simulink model "CM13_2024a_MachE_for_UA_HIL"  (R2024a)
settings: Solver=ode1  StartTime=0.0  StopTime=Inf  FixedStep=0.001  RelTol=1e-3  EnableMultiTasking=on
PreLoadFcn:
  | % if ~length(which('cmcmd')), cmenv; end
PostLoadFcn:
  | if any(exist('dsrtsu_mdlpostloadfcn', 'file') ~= 0), dsrtsu_mdlpostloadfcn('Execute', bdroot); end
InitFcn:
  | , if any(exist('rtifpga_mdlclblib', 'file') ~= 0), rtifpga_mdlclblib('Init', bdroot); end,
  | , if any(exist('dsmpb_private', 'file') ~= 0), dsmpb_private('dsmpb_mdlclblib', 'Init', bdroot); end,
values from neighbouring files (symbols this model uses):
  CoastDown =     [Run_Simulink.mat]
  limitedMCT =     [Run_Simulink.mat]
  MCT =     [Run_Simulink.mat]
  pMCT =     [Run_Simulink.mat]
  RealSimPara =     [Run_Simulink.mat]
  Ref_speed = [13 13.007895099 13.015778396 13.023649891 13.031509584 13.039357475 13.047193564 13.055017851 13.062830336 13.070631019 13.0784199 13.086196979 ... (2669 elements, 2669x1)]    [Ref_speed_and_time.mat]
  Ref_time = [0 0.01 0.02 0.03 0.04 0.05 0.06 0.07 0.08 0.09 0.1 0.11 ... (2669 elements, 2669x1)]    [Ref_speed_and_time.mat]
  US06 =     [Run_Simulink.mat]
undefined symbols (not defined in the file or in its folder): AccelCmd, ActTqLF_Nm_, ActTqLR_Nm_, ActTqRF_Nm_, ActTqRR_Nm_, BattChargeLimitMaxPwr, BattChargeLimitSocBpts, BattChargeLimitTbl, BattChrgCapcty, BattDischargeLimitSocBpts, BattDischargeLimitTbl, BattDischargeMaxPwr, BattNumCellsParallel, BattNumCellsSeries, BattOpenVoltCapBpts, BattOpenVoltTbl, BattResistSocBpts, BattResistTbl, BattResistTempBpts, BrakeMaxPrs, BrakeMaxTrq, ChassisDistCg2FrontAxle, ChassisDistCg2RearAxle, ChassisVehMass, CltchCmd, DecelCmd, DiffRatio, DiscIntNeverNeededParam, EnvGravCnst, EnvPrs, EnvTemp, FuelSpecificGrav, GearCmd, h, InitStates, lgSw, MtrEffSpdBpts, MtrEffTbl, MtrEffTrqBpts, MtrPwrMax, MtrTrqMax, planned_speed, planned_time, ref_speed, ref_time, rticanmm_blockfcn, rticanmm_initfcn, SteeringCmd, SupvsryCtrlRegenBrkCutOffTbl, SupvsryCtrlRegenSpdBpts, TestScnrioCycleNum, VEH
libraries: simulink x264, VSIGenLib x262, etargetslib x201, dsmpblib x161, CarMaker4SL x142, rtimmsu_dsrtlib x32, vehdynlibtire x24, autolibshared x19, vehdynlibsuspension x14, vehdynlibtirecommon x14, autolibutils x10, VsrLibWheel x8
(part 16 of 48)

== system CM13_2024a_MachE_for_UA_HIL/CarMaker_new/IPG Vehicle/Driver and Drive Cycle/Get Cycle Clock Time ==
  Cycle Trigger : Inport
  Add1 : Sum  Inputs=+-
  Clock1 : Clock
  Clock2 : Clock
  Data Type Conversion : DataTypeConversion  OutDataTypeStr=double  SaturateOnIntegerOverflow=off  RndMeth=Floor
  Memory4 : Memory
  Switch : Switch  Criteria=u2 > Threshold  SaturateOnIntegerOverflow=off  InputSameDT=off
  tCycle : Outport
  wires:
  Switch/1 -> Add1/2, Memory4/1
  Clock1/1 -> Add1/1
  Clock2/1 -> Switch/3
  Add1/1 -> tCycle/1  "tCycle"
  Memory4/1 -> Switch/1
  Cycle Trigger/1 -> Data Type Conversion/1
  Data Type Conversion/1 -> Switch/2

== system CM13_2024a_MachE_for_UA_HIL/CarMaker_new/IPG Vehicle/Driver and Drive Cycle/IDM ==
  note: In IPG, when the ego vehicle slipped side to side, it will ignore the front vehicle as in the path. The <RadarL> "detects nearest point in the path" , thus ego vehilce will no longer consider the front vehilce as "in path" and ACC/IDM will have incorrect output.
      |
      | Second object sensor <Backup> is added, it dectects nearest point, ensuring ego vehicle stopped at close range.
  CM_Time : Inport
  Add1 : Sum
  Add2 : Sum
  Add3 : Sum  Commented=on
  Bus Selector : BusSelector  OutputSignals=NearPnt ds x,NearPnt ds y,NearPnt dv x
  Bus Selector1 : BusSelector  OutputSignals=dtct
  Bus Selector2 : BusSelector  OutputSignals=dtct
  Bus Selector3 : BusSelector  OutputSignals=NearPnt ds x,NearPnt ds y
  Bus Selector4 : BusSelector  Commented=on  OutputSignals=NearPnt ds x,NearPnt ds y,NearPnt dv x
  Bus Selector5 : BusSelector  Commented=on  OutputSignals=dtct
  Bus Selector6 : BusSelector  OutputSignals=Dist,Vrel
  Compare To Constant : simulink/Logic and Bit Operations/Compare To Constant  relop=>=  const=30  OutDataTypeStr=boolean
  Constant : Constant  Value=0
  Constant1 : Constant  Value=99999
  Constant2 : Constant  Value=99999
  Dis2lead_Raw : Scope
  Math Function{,1..3} (4 alike) : Math  Operator=square
  Math Function4 : Math  Commented=on  Operator=square
  Math Function5 : Math  Commented=on  Operator=square
  ObjIndex : Scope
  Object Sensor 1 : CarMaker4SL/Sensors/Object Sensor  xname=RadarS  xstime=Continuous
      settings: SourceProductName=CarMaker4SL
  Object Sensor 2 : CarMaker4SL/Sensors/Object Sensor  xname=RadarL  xstime=Continuous
      settings: SourceProductName=CarMaker4SL
  Object Sensor Object : CarMaker4SL/Sensors/Object Sensor Object  Commented=on  xname=RadarL  ximode=Observed Objects  xstime=Continuous
      settings: SourceProductName=CarMaker4SL
  Object Sensor Object 1 : CarMaker4SL/Sensors/Object Sensor Object  xname=INPORT  ximode=Observed Objects  xstime=Continuous
      settings: SourceProductName=CarMaker4SL
  Object Sensor Object 2 : CarMaker4SL/Sensors/Object Sensor Object  xname=INPORT  ximode=Observed Objects  xstime=Continuous
      settings: SourceProductName=CarMaker4SL
  Radar Sensor : CarMaker4SL/Sensors/Radar Sensor  xname=RadarReal  xstime=Continuous
      settings: SourceProductName=CarMaker4SL
  Radar Sensor Object : CarMaker4SL/Sensors/Radar Sensor Object  xname=INPORT  ximode=Observed Objects  xstime=Continuous
      settings: SourceProductName=CarMaker4SL
  Read CM Dict1 : CarMaker4SL/Read CM Dict  xname=Car.v  xsync=off  xstime=Continuous
  Scope1 : Scope  Commented=on
  Scope2 : Scope  Commented=on
  Scope3 : Scope
  Scope4 : Scope
  Square Root : Sqrt
  Square Root1 : Sqrt
  Square Root2 : Sqrt  Commented=on
  Subsystem : Subsystem
  Switch1 : Switch  Criteria=u2 > Threshold  SaturateOnIntegerOverflow=off  InputSameDT=off
  ego_ref_spd_m/s : Outport
  wires:
  Add1/1 -> Square Root/1
  Bus Selector1/1 -> Subsystem/1(is_detected)  "<dtct>"
  Bus Selector/3 -> Subsystem/4(rel_front_spd_m/s)  "<NearPnt dv x>"
  Object Sensor Object 2/3 -> Bus Selector1/1
  Read CM Dict1/1 -> Subsystem/2(ego_spd_m/s)  "VehSpd"
  Math Function/1 -> Add1/1
  Object Sensor Object 2/5 -> Bus Selector/1
  Math Function1/1 -> Add1/2
  Object Sensor 2/1 -> Object Sensor Object 2/1
  Constant2/1 -> Object Sensor Object 2/2
  Bus Selector/1 -> Math Function/1  "<NearPnt ds x>"
  Bus Selector/2 -> Math Function1/1  "<NearPnt ds y>"
  Subsystem/1(ego_ref_spd_m/s) -> Switch1/1
  Object Sensor 1/1 -> Object Sensor Object 1/1
  Constant1/1 -> Object Sensor Object 1/2
  Object Sensor Object 1/3 -> Bus Selector2/1
  Bus Selector2/1 -> Subsystem/5(backup_detected)  "<dtct>"
  CM_Time/1 -> [CM_Time]
  Compare To Constant/1 -> Switch1/2
  Constant/1 -> Switch1/3
  Switch1/1 -> ego_ref_spd_m/s/1
  [CM_Time] -> Compare To Constant/1
  Object Sensor Object 1/5 -> Bus Selector3/1
  Math Function3/1 -> Add2/2
  Math Function2/1 -> Add2/1
  Add2/1 -> Square Root1/1
  Bus Selector3/1 -> Math Function2/1  "<NearPnt ds x>"
  Bus Selector3/2 -> Math Function3/1  "<NearPnt ds y>"
  Bus Selector4/2 -> Math Function5/1  "<NearPnt ds y>"
  Bus Selector4/1 -> Math Function4/1  "<NearPnt ds x>"
  Object Sensor Object/3 -> Bus Selector5/1
  Object Sensor Object/5 -> Bus Selector4/1
  Square Root2/1 -> Scope1/1
  Bus Selector4/3 -> Scope2/1  "<NearPnt dv x>"
  Add3/1 -> Square Root2/1
  Math Function4/1 -> Add3/1
  Math Function5/1 -> Add3/2
  Square Root1/1 -> Subsystem/6(front_obj_dist_m)
  Square Root/1 -> Subsystem/3(int_veh_dist_m), Dis2lead_Raw/1
  Radar Sensor/1 -> Radar Sensor Object/1
  Radar Sensor Object/2 -> Bus Selector6/1
  Bus Selector6/1 -> Scope3/1  "<Dist>"
  Bus Selector6/2 -> Scope4/1  "<Vrel>"
  Object Sensor Object 2/1 -> ObjIndex/1

== system CM13_2024a_MachE_for_UA_HIL/CarMaker_new/IPG Vehicle/Mach-E CAN BM/Subsystem ==
  note: softRCM ECU
  Bus Creator : BusCreator  Inputs=5
  Logic : Subsystem
  Noise Generators : Subsystem  Commented=on
  Read CM Dict : CarMaker4SL/Read CM Dict  xname=Car.RollVel  xsync=off  xstime=Continuous
  Read CM Dict1 : CarMaker4SL/Read CM Dict  xname=Car.YawRate  xsync=off  xstime=Continuous
  Read CM Dict2 : CarMaker4SL/Read CM Dict  xname=Car.ax  xsync=off  xstime=Continuous
  Read CM Dict3 : CarMaker4SL/Read CM Dict  xname=Car.ay  xsync=off  xstime=Continuous
  Read CM Dict4 : CarMaker4SL/Read CM Dict  xname=Car.az  xsync=off  xstime=Continuous
  AccelYaw_out : Outport
  wires:
  Logic/1(Out1) -> AccelYaw_out/1
  Bus Creator/1 -> Logic/1(In1)
  Read CM Dict4/1 -> Bus Creator/5  "a_z_Vehicle_CoG_withG[m|s2]"
  Read CM Dict3/1 -> Bus Creator/4  "a_y_Vehicle_CoG_withG[m|s2]"
  Read CM Dict2/1 -> Bus Creator/3  "a_x_Vehicle_CoG_withG[m|s2]"
  Read CM Dict/1 -> Bus Creator/1  "RollRate_Vehicle_CoG[rad|s]"
  Read CM Dict1/1 -> Bus Creator/2  "YawRate_Vehicle_CoG[rad|s]"

== system CM13_2024a_MachE_for_UA_HIL/CarMaker_new/IPG Vehicle/Mach-E CAN BM/Subsystem1 ==
  note: softRCM ECU
  Roll : Inport
  Yaw : Inport  Port=2
  A_x : Inport  Port=3
  A_y : Inport  Port=4
  A_z : Inport  Port=5
  Add{,1..4} (5 alike) : Sum
  Bus Creator : BusCreator  Inputs=5
  Logic : Subsystem
  Noise Generators : Subsystem  Commented=on
  Read CM Dict : CarMaker4SL/Read CM Dict  xname=Car.RollVel  xsync=off  xstime=Continuous
  Read CM Dict1 : CarMaker4SL/Read CM Dict  xname=Car.YawRate  xsync=off  xstime=Continuous
  Read CM Dict2 : CarMaker4SL/Read CM Dict  xname=Car.ax  xsync=off  xstime=Continuous
  Read CM Dict3 : CarMaker4SL/Read CM Dict  xname=Car.ay  xsync=off  xstime=Continuous
  Read CM Dict4 : CarMaker4SL/Read CM Dict  xname=Car.az  xsync=off  xstime=Continuous
  AccelYaw_out : Outport
  wires:
  Add/1 -> Bus Creator/5  "a_z_Vehicle_CoG_withG[m|s2]"
  Add2/1 -> Bus Creator/3  "a_x_Vehicle_CoG_withG[m|s2]"
  Add4/1 -> Bus Creator/2  "YawRate_Vehicle_CoG[rad|s]"
  Add1/1 -> Bus Creator/4  "a_y_Vehicle_CoG_withG[m|s2]"
  Add3/1 -> Bus Creator/1  "RollRate_Vehicle_CoG[rad|s]"
  Logic/1(Out1) -> AccelYaw_out/1
  Bus Creator/1 -> Logic/1(In1)
  Read CM Dict4/1 -> Add/1  "a_z_Vehicle_CoG_withG[m|s2]"
  Read CM Dict3/1 -> Add1/1  "a_y_Vehicle_CoG_withG[m|s2]"
  Read CM Dict2/1 -> Add2/1  "a_x_Vehicle_CoG_withG[m|s2]"
  Read CM Dict/1 -> Add3/1  "RollRate_Vehicle_CoG[rad|s]"
  Read CM Dict1/1 -> Add4/1  "YawRate_Vehicle_CoG[rad|s]"
  Yaw/1 -> Add4/2
  A_x/1 -> Add2/2
  A_y/1 -> Add1/2
  Roll/1 -> Add3/2
  A_z/1 -> Add/2

== system CM13_2024a_MachE_for_UA_HIL/CarMaker_new/IPG Vehicle/MachE CAN/RTICANMM Gateway ==
  Enable : Inport
  DSRT Data Hook1 : rtimmsu_dsrtlib/Data Hook  ControllerName=RCM_ECU  PortID=RTICANMMRCM_ECU  BlockSet=can  blockdata=struct('version','1.0')
  DSRT Data Hook2 : rtimmsu_dsrtlib/Data Hook  ControllerName=RCM_Harness  PortID=RTICANMMRCM_Harness  BlockSet=can  blockdata=struct('version','1.0')
  ModelClose : Subsystem  mask(RTICANMMModelClose){}
  TRC Exclusion : rtimmsu_dsrtlib/TRC Exclusion
  sfcn : S-Function  InitFcn=rticanmm_initfcn(gcb, 'SFCNs')  FunctionName=RTICANMM_GW_RCM_Gateway  SFunctionDeploymentMode=off  EnableBusSupport=off
      mask init:
      | rticanmm_initfcn(gcb, 'SFCNs')
  Bus1TXCounter : Outport  VectorParamsAs1DForOutWhenUnconnected=off
  Bus1RXCounter : Outport  Port=2  VectorParamsAs1DForOutWhenUnconnected=off
  Bus2TXCounter : Outport  Port=3  VectorParamsAs1DForOutWhenUnconnected=off
  Bus2RXCounter : Outport  Port=4  VectorParamsAs1DForOutWhenUnconnected=off
  wires:
  Enable/1 -> sfcn/1
  sfcn/1 -> Bus1TXCounter/1
  sfcn/2 -> Bus1RXCounter/1
  sfcn/3 -> Bus2TXCounter/1
  sfcn/4 -> Bus2RXCounter/1

== system CM13_2024a_MachE_for_UA_HIL/CarMaker_new/IPG Vehicle/MachE CAN/RTICANMM GeneralSetup ==
  Constant : Constant
  ModelClose : Subsystem  mask(RTICANMMModelClose){}
  TRC Exclusion : rtimmsu_dsrtlib/TRC Exclusion
  Terminator : Terminator
  wires:
  Constant/1 -> Terminator/1

== system CM13_2024a_MachE_for_UA_HIL/CarMaker_new/IPG Vehicle/MachE CAN/RTICANMM MachE_HS1 ==
  VariationInput : Inport
  Reset : Inport  Port=2
  DSRT Data Hook : rtimmsu_dsrtlib/Data Hook  ControllerName=MachE_HS1  PortID=RTICANMMMachE_HS1  BlockSet=RTICANMM  blockdata=struct('version','1.0')  MMType=ControllerSetup
  ModelClose : Subsystem  mask(RTICANMMModelClose){}
  RTICANMMCHANNEL_TLC : S-Function  FunctionName=rticanmm_tlc_adv  Parameters='DSRT',-1,-1,-1,500,26711143421  SFunctionDeploymentMode=off  EnableBusSupport=off  mask(RTICANMMCHANNEL_TLC){}
  Variation_DTC : DataTypeConversion
  sfcn : S-Function  InitFcn=rticanmm_initfcn(gcb, 'SFCNs')  FunctionName=RTICANMM_SETUP_MachE_HS1  SFunctionDeploymentMode=off  EnableBusSupport=off
      mask init:
      | rticanmm_initfcn(gcb, 'SFCNs')
  wires:
  Reset/1 -> sfcn/2
  VariationInput/1 -> Variation_DTC/1
  Variation_DTC/1 -> sfcn/1

== system CM13_2024a_MachE_for_UA_HIL/CarMaker_new/IPG Vehicle/MachE CAN/RTICANMM MainBlock ==
  DSRT Data Hook : rtimmsu_dsrtlib/Data Hook  ControllerName=RCM_ECU  PortID=RTICANMMRCM_ECU  BlockSet=RTICANMM  blockdata=struct('version','1.0')  Variant=RCM_ECU  MMType=mainsetup
  ModelClose : Subsystem  mask(RTICANMMModelClose){}
  TRC Exclusion : rtimmsu_dsrtlib/TRC Exclusion
  converter : Subsystem  mask(CANnedyVector2Bus){}
      mask help: Do not change.
      mask Display: disp('Vector to\nBus')
  sfcn : S-Function  InitFcn=rticanmm_initfcn(gcb, 'SFCNs')  FunctionName=RTICANMM_MAIN_RCM_ECU  SFunctionDeploymentMode=off  EnableBusSupport=off
      mask init:
      | rticanmm_initfcn(gcb, 'SFCNs')
  RX_Data : Outport
  wires:
  converter/1(out) -> RX_Data/1
  sfcn/1 -> converter/1(in_1)
  sfcn/2 -> converter/2(in_2)
  sfcn/3 -> converter/3(in_3)
  sfcn/4 -> converter/4(in_4)
  sfcn/5 -> converter/5(in_5)
  sfcn/6 -> converter/6(in_6)
  sfcn/7 -> converter/7(in_7)
  sfcn/8 -> converter/8(in_8)
  sfcn/9 -> converter/9(in_9)
  sfcn/10 -> converter/10(in_10)
  sfcn/11 -> converter/11(in_11)
  sfcn/12 -> converter/12(in_12)
  sfcn/13 -> converter/13(in_13)
  sfcn/14 -> converter/14(in_14)

== system CM13_2024a_MachE_for_UA_HIL/CarMaker_new/IPG Vehicle/MachE CAN/RTICANMM MainBlock1 ==
  TXData : Inport
  DSRT Data Hook : rtimmsu_dsrtlib/Data Hook  ControllerName=RCM_Harness  PortID=RTICANMMRCM_Harness  BlockSet=RTICANMM  blockdata=struct('version','1.0')  Variant=RCM_Harness  MMType=mainsetup
  ModelClose : Subsystem  mask(RTICANMMModelClose){}
  TRC Exclusion : rtimmsu_dsrtlib/TRC Exclusion
  TXINselector1 : BusSelector  OutputSignals=Accel_Data.VehLatLongVert_No_Cnt,Accel_Data.VehLatLongVertA_No_Cs,Accel_Data.VehVert2_A_Actl,Accel_Data.VehVertAActl_D_Qf,Accel_Data.VehLong2_A_Actl,Accel_Data.VehLongAActl_D_Qf,Accel_Data.VehLat2_A_Actl,Accel_Data.VehLatAActl_D_Qf,Yaw_Data.VehYawWActl_D_Qf,Yaw_Data.VehRolWActl_D_Qf,Yaw_Data.VehRollYaw_No_Cnt,Yaw_Data.VehRollYawW_No_Cs,Yaw_Data.VehYaw_W_Actl,Yaw_Data.VehRol_W_Actl
  converter : Subsystem  mask(CANnedyVector2Bus){}
      mask help: Do not change.
      mask Display: disp('Vector to\nBus')
  sfcn : S-Function  InitFcn=rticanmm_initfcn(gcb, 'SFCNs')  FunctionName=RTICANMM_MAIN_RCM_Harness  SFunctionDeploymentMode=off  EnableBusSupport=off
      mask init:
      | rticanmm_initfcn(gcb, 'SFCNs')
  RX_Data : Outport
  wires:
  TXData/1 -> TXINselector1/1
  TXINselector1/1 -> sfcn/1  "<VehLatLongVert_No_Cnt>"
  TXINselector1/2 -> sfcn/2  "<VehLatLongVertA_No_Cs>"
  TXINselector1/3 -> sfcn/3  "<VehVert2_A_Actl>"
  TXINselector1/4 -> sfcn/4  "<VehVertAActl_D_Qf>"
  TXINselector1/5 -> sfcn/5  "<VehLong2_A_Actl>"
  TXINselector1/6 -> sfcn/6  "<VehLongAActl_D_Qf>"
  TXINselector1/7 -> sfcn/7  "<VehLat2_A_Actl>"
  TXINselector1/8 -> sfcn/8  "<VehLatAActl_D_Qf>"
  TXINselector1/9 -> sfcn/9  "<VehYawWActl_D_Qf>"
  TXINselector1/10 -> sfcn/10  "<VehRolWActl_D_Qf>"
  TXINselector1/11 -> sfcn/11  "<VehRollYaw_No_Cnt>"
  TXINselector1/12 -> sfcn/12  "<VehRollYawW_No_Cs>"
  TXINselector1/13 -> sfcn/13  "<VehYaw_W_Actl>"
  TXINselector1/14 -> sfcn/14  "<VehRol_W_Actl>"
  converter/1(out) -> RX_Data/1
  sfcn/1 -> converter/1(in_1)

== system CM13_2024a_MachE_for_UA_HIL/CarMaker_new/IPG Vehicle/MachE CAN/RTICANMM MainBlock2 ==
  TXData : Inport
  DSRT Data Hook : rtimmsu_dsrtlib/Data Hook  ControllerName=MachE_HS1  PortID=RTICANMMMachE_HS1  BlockSet=RTICANMM  blockdata=struct('version','1.0')  Variant=MachE_HS1  MMType=mainsetup
  ModelClose : Subsystem  mask(RTICANMMModelClose){}
  TRC Exclusion : rtimmsu_dsrtlib/TRC Exclusion
  TXINselector1 : BusSelector  OutputSignals=Gear_Shift_by_Wire_3_HS1.TrnGear_D_RqPt
  sfcn : S-Function  InitFcn=rticanmm_initfcn(gcb, 'SFCNs')  FunctionName=RTICANMM_MAIN_MachE_HS1  SFunctionDeploymentMode=off  EnableBusSupport=off
      mask init:
      | rticanmm_initfcn(gcb, 'SFCNs')
  wires:
  TXData/1 -> TXINselector1/1
  TXINselector1/1 -> sfcn/1  "<TrnGear_D_RqPt>"

== system CM13_2024a_MachE_for_UA_HIL/CarMaker_new/IPG Vehicle/MachE CAN/RTICANMM RCM_ECU ==
  VariationInput : Inport
  Reset : Inport  Port=2
  DSRT Data Hook : rtimmsu_dsrtlib/Data Hook  ControllerName=RCM_ECU  PortID=RTICANMMRCM_ECU  BlockSet=RTICANMM  blockdata=struct('version','1.0')  MMType=ControllerSetup
  ModelClose : Subsystem  mask(RTICANMMModelClose){}
  RTICANMMCHANNEL_TLC : S-Function  FunctionName=rticanmm_tlc_adv  Parameters='DSRT',-1,-1,-1,500,26711143421  SFunctionDeploymentMode=off  EnableBusSupport=off  mask(RTICANMMCHANNEL_TLC){}
  Variation_DTC : DataTypeConversion
  sfcn : S-Function  InitFcn=rticanmm_initfcn(gcb, 'SFCNs')  FunctionName=RTICANMM_SETUP_RCM_ECU  SFunctionDeploymentMode=off  EnableBusSupport=off
      mask init:
      | rticanmm_initfcn(gcb, 'SFCNs')
  wires:
  Reset/1 -> sfcn/2
  VariationInput/1 -> Variation_DTC/1
  Variation_DTC/1 -> sfcn/1

== system CM13_2024a_MachE_for_UA_HIL/CarMaker_new/IPG Vehicle/MachE CAN/RTICANMM RCM_Harness ==
  VariationInput : Inport
  Reset : Inport  Port=2
  DSRT Data Hook : rtimmsu_dsrtlib/Data Hook  ControllerName=RCM_Harness  PortID=RTICANMMRCM_Harness  BlockSet=RTICANMM  blockdata=struct('version','1.0')  MMType=ControllerSetup
  ModelClose : Subsystem  mask(RTICANMMModelClose){}
  RTICANMMCHANNEL_TLC : S-Function  FunctionName=rticanmm_tlc_adv  Parameters='DSRT',-1,-1,-1,500,26711143421  SFunctionDeploymentMode=off  EnableBusSupport=off  mask(RTICANMMCHANNEL_TLC){}
  Variation_DTC : DataTypeConversion
  sfcn : S-Function  InitFcn=rticanmm_initfcn(gcb, 'SFCNs')  FunctionName=RTICANMM_SETUP_RCM_Harness  SFunctionDeploymentMode=off  EnableBusSupport=off
      mask init:
      | rticanmm_initfcn(gcb, 'SFCNs')
  BUS_STATE : Outport
  STATUS_STUFF_BIT_ERROR : Outport  Port=2
  STATUS_FORM_ERROR : Outport  Port=3
  STATUS_CRC_ERROR : Outport  Port=4
  STATUS_LOST_RX_NUM : Outport  Port=5
  STATUS_REC_RX_NUM : Outport  Port=6
  STATUS_SENT_TX_NUM : Outport  Port=7
  wires:
  Reset/1 -> sfcn/2
  sfcn/1 -> BUS_STATE/1
  sfcn/2 -> STATUS_STUFF_BIT_ERROR/1
  sfcn/3 -> STATUS_FORM_ERROR/1
  sfcn/4 -> STATUS_CRC_ERROR/1
  sfcn/5 -> STATUS_LOST_RX_NUM/1
  sfcn/6 -> STATUS_REC_RX_NUM/1
  sfcn/7 -> STATUS_SENT_TX_NUM/1
  VariationInput/1 -> Variation_DTC/1
  Variation_DTC/1 -> sfcn/1

== system CM13_2024a_MachE_for_UA_HIL/CarMaker_new/IPG Vehicle/MachE CAN/Subsystem ==
  note: softRCM ECU
  Roll : Inport
  Yaw : Inport  Port=2
  A_x : Inport  Port=3
  A_y : Inport  Port=4
  A_z : Inport  Port=5
  Add{,1..4} (5 alike) : Sum
  Bus Creator : BusCreator  Inputs=5
  Logic : Subsystem
  Mapping : Subsystem
  Noise Generators : Subsystem  Commented=on
  Read CM Dict : CarMaker4SL/Read CM Dict  xname=Car.RollVel  xsync=off  xstime=Continuous
  Read CM Dict1 : CarMaker4SL/Read CM Dict  xname=Car.YawRate  xsync=off  xstime=Continuous
  Read CM Dict2 : CarMaker4SL/Read CM Dict  xname=Car.ax  xsync=off  xstime=Continuous
  Read CM Dict3 : CarMaker4SL/Read CM Dict  xname=Car.ay  xsync=off  xstime=Continuous
  Read CM Dict4 : CarMaker4SL/Read CM Dict  xname=Car.az  xsync=off  xstime=Continuous
  Accel_Data_out : Outport
  Yaw_Data_out : Outport  Port=2
  wires:
  Add/1 -> Bus Creator/5  "a_z_Vehicle_CoG_withG[m|s2]"
  Add2/1 -> Bus Creator/3  "a_x_Vehicle_CoG_withG[m|s2]"
  Add4/1 -> Bus Creator/2  "YawRate_Vehicle_CoG[rad|s]"
  Add1/1 -> Bus Creator/4  "a_y_Vehicle_CoG_withG[m|s2]"
  Add3/1 -> Bus Creator/1  "RollRate_Vehicle_CoG[rad|s]"
  Logic/1(Out1) -> Mapping/1(In1)
  Bus Creator/1 -> Logic/1(In1)
  Read CM Dict4/1 -> Add/1  "a_z_Vehicle_CoG_withG[m|s2]"
  Read CM Dict3/1 -> Add1/1  "a_y_Vehicle_CoG_withG[m|s2]"
  Read CM Dict2/1 -> Add2/1  "a_x_Vehicle_CoG_withG[m|s2]"
  Read CM Dict/1 -> Add3/1  "RollRate_Vehicle_CoG[rad|s]"
  Read CM Dict1/1 -> Add4/1  "YawRate_Vehicle_CoG[rad|s]"
  Mapping/1(Accel_Data_Out) -> Accel_Data_out/1  "MsgSignals"
  Mapping/2(Yaw_Data_Out) -> Yaw_Data_out/1
  Yaw/1 -> Add4/2
  A_x/1 -> Add2/2
  A_y/1 -> Add1/2
  Roll/1 -> Add3/2
  A_z/1 -> Add/2

== system CM13_2024a_MachE_for_UA_HIL/CarMaker_new/IPG Vehicle/MachE CAN/User2RTICANMM MainBlock1 ==
  "Accel_Data " : Inport
  Yaw : Inport  Port=2
  Accel_Data : Subsystem
  Yaw_Data : Subsystem
  buscreator : BusCreator  Inputs=2
  out : Outport
  wires:
  Accel_Data/1(out) -> buscreator/1  "Accel_Data"
  Yaw_Data/1(out) -> buscreator/2  "Yaw_Data"
  buscreator/1 -> out/1  "CAN"
  "Accel_Data "/1 -> Accel_Data/1(Input)
  Yaw/1 -> Yaw_Data/1(Input)

== system CM13_2024a_MachE_for_UA_HIL/CarMaker_new/IPG Vehicle/MachE CAN/User2RTICANMM MainBlock2 ==
  Gear_Shift_by_Wire_3_HS1 : Subsystem
  buscreator : BusCreator  Inputs=1
  out : Outport
  wires:
  Gear_Shift_by_Wire_3_HS1/1(out) -> buscreator/1  "Gear_Shift_by_Wire_3_HS1"
  buscreator/1 -> out/1  "CAN"

== system CM13_2024a_MachE_for_UA_HIL/CarMaker_new/IPG Vehicle/Rototest and ORNL Interface/DummyPT ==
  WhlSpeedIn : Inport
  APPToTorque : Lookup_n-D  NumberOfTableDimensions=1  BreakpointsForDimension1=[0 100]  Table=[0 184]  InternalRulePriority=Speed  RndMeth=Simplest
  APPToTorque1 : Lookup_n-D  NumberOfTableDimensions=1  BreakpointsForDimension1=[0 100]  Table=[0 184]  InternalRulePriority=Speed  RndMeth=Simplest
  APP_pct : Constant  Value=0
  BPP_pct : Constant  Value=0
  FDR : Gain  Gain=3.18
  Flip : Gain  Gain=-1
  Gear : Product
  Memory : Memory
  NissanTrans : Lookup_n-D  NumberOfTableDimensions=1  BreakpointsForDimension1=[0 5 10 15 25 34 45 55]  Table=[5.25 3.03 1.95 1.46 1.22 1.00 0.81 0.67]  ExtrapMethod=Clip  InternalRulePriority=Speed  RndMeth=Simplest
  Sum : Sum  Inputs=++|
  WheelRadius : Gain  Gain=0.3235
  kph2mph : Gain  Gain=0.621
  mps2kph : Gain  Gain=3.6
  WheelTorqueOut : Outport
  wires:
  kph2mph/1 -> NissanTrans/1  "Speed_mph"
  APPToTorque/1 -> Sum/1  "APPTorque"
  mps2kph/1 -> kph2mph/1  "Speed_kph"
  BPP_pct/1 -> APPToTorque1/1
  NissanTrans/1 -> Gear/2  "Gear"
  Gear/1 -> FDR/1  "TransTorqueOut"
  APPToTorque1/1 -> Flip/1
  Flip/1 -> Sum/2  "BPPTorque"
  APP_pct/1 -> APPToTorque/1
  Sum/1 -> Gear/1  "TorqueTotal"
  WheelRadius/1 -> mps2kph/1  "Speed_mps"
  FDR/1 -> Memory/1  "WheelTorqueOut"
  WhlSpeedIn/1 -> WheelRadius/1
  Memory/1 -> WheelTorqueOut/1

== system CM13_2024a_MachE_for_UA_HIL/CarMaker_new/IPG Vehicle/Rototest and ORNL Interface/Format CM Powertrain Signals ==
  note: Can Bypass with my own brake model
  BrakingTorques : Inport
  RotoWheelSpd : Inport  Port=2
  AxlTrq : Inport  Port=3
  MaxRegen : Inport  Port=4
  Bus Creator1 : BusCreator  Inputs=42
  Bus Selector2 : BusSelector  OutputSignals=Brake IF Trq_WB FL,Brake IF Trq_WB FR,Brake IF Trq_WB RL,Brake IF Trq_WB RR
  BusCreator2 : BusCreator  Inputs=42
  Demux : Demux
  Demux1 : Demux  Outputs=42
      settings: DisplayOption=none
  Demux2 : Demux
  Discrete-Time Integrator{4..7} (4 alike) : DiscreteIntegrator  IntegratorMethod=Integration: Backward Euler  SampleTime=0.001  ICPrevOutput=DiscIntNeverNeededParam  ICPrevScaledInput=DiscIntNeverNeededParam
  Gain{5..8} (4 alike) : Gain  Gain=-1
  Ground{2..5} (4 alike) : Ground
  Ignition : Constant
  Memory{1..4} (4 alike) : Memory
  Operation Error : Constant  Value=4
  Operation State Driving : Constant  Value=4
  Product{1..4} (4 alike) : Product  RndMeth=Zero
  Saturation{1..4} (4 alike) : Saturate  UpperLimit=1  LowerLimit=-1
  Zero{1..5} (5 alike) : Constant  Value=0
  PowerTrainOutIdeal : Outport
  wires:
  Saturation4/1 -> Product4/2
  Demux1/3 -> BusCreator2/3  "PT IF OperationError"
  Demux1/2 -> BusCreator2/2  "PT IF OperationState"
  Demux1/40 -> BusCreator2/40  "PT IF WRR Trq_Supp2WC"
  Demux1/9 -> BusCreator2/9  "PT IF Trq_Supp2Bdy1B x"
  Discrete-Time Integrator6/1 -> Bus Creator1/29  "PT WRL rot"
  Demux1/1 -> BusCreator2/1  "PT IF Ignition"
  MaxRegen/1 -> Bus Creator1/28, Bus Creator1/21
  BusCreator2/1 -> PowerTrainOutIdeal/1
  Operation State Driving/1 -> Bus Creator1/2
  Gain8/1 -> Bus Creator1/38
  Demux1/16 -> BusCreator2/16  "PT IF WFL rotv"
  Demux1/21 -> BusCreator2/21  "PT IF WFL Trq_BrakeReg_max"
  Ground2/1 -> Bus Creator1/7
  Demux1/23 -> BusCreator2/23  "PT IF WFR rotv"
  Demux1/14 -> BusCreator2/14  "PT IF DL_iDiff_mean"
  Demux1/4 -> BusCreator2/4  "PT IF GearNo"
  Demux1/17 -> BusCreator2/17  "PT IF WFL Trq_B2W"
  Product3/1 -> Gain5/1
  Demux1/5 -> BusCreator2/5  "PT IF Engine_rotv"
  Demux1/11 -> BusCreator2/11  "PT IF Trq_Supp2Bdy1B z"
  Demux1/12 -> BusCreator2/12  "PT IF Trq_Supp2BdyEng x"
  Demux1/7 -> BusCreator2/7  "PT IF Trq_Supp2Bdy1 y"
  Discrete-Time Integrator5/1 -> Bus Creator1/22  "PT WFR rot"
  Demux1/42 -> BusCreator2/42  "PT IF WRR Trq_BrakeReg_max"
  Gain5/1 -> Bus Creator1/17
  Demux1/18 -> BusCreator2/18  "PT IF WFL Trq_Drive"
  Demux1/8 -> BusCreator2/8  "PT IF Trq_Supp2Bdy1 z"
  Demux1/38 -> BusCreator2/38  "PT IF WRR Trq_B2W"
  Memory4/1 -> Saturation4/1
  Demux1/10 -> BusCreator2/10  "PT IF Trq_Supp2Bdy1B y"
  Demux1/27 -> BusCreator2/27  "PT IF WFR Trq_BrakeReg"
  Demux1/24 -> BusCreator2/24  "PT IF WFR Trq_B2W"
  Demux1/25 -> BusCreator2/25  "PT IF WFR Trq_Drive"
  Demux1/26 -> BusCreator2/26  "PT IF WFR Trq_Supp2WC"
  Demux1/13 -> BusCreator2/13  "PT IF Trq_Supp2BdyEng y"
  Demux1/15 -> BusCreator2/15  "PT IF WFL rot"
  Bus Selector2/2 -> Product1/1  "<Brake IF Trq_WB FR>"
  Memory3/1 -> Saturation3/1
  Demux1/19 -> BusCreator2/19  "PT IF WFL Trq_Supp2WC"
  Demux1/22 -> BusCreator2/22  "PT IF WFR rot"
  Demux1/29 -> BusCreator2/29  "PT IF WRL rot"
  Demux1/33 -> BusCreator2/33  "PT IF WRL Trq_Supp2WC"
  Demux1/30 -> BusCreator2/30  "PT IF WRL rotv"
  Demux1/28 -> BusCreator2/28  "PT IF WFR Trq_BrakeReg_max"
  Demux1/35 -> BusCreator2/35  "PT IF WRL Trq_BrakeReg_max"
  Demux1/39 -> BusCreator2/39  "PT IF WRR Trq_Drive"
  Zero4/1 -> Bus Creator1/33, Bus Creator1/34, Bus Creator1/35
  Demux1/34 -> BusCreator2/34  "PT IF WRL Trq_BrakeReg"
  Demux1/37 -> BusCreator2/37  "PT IF WRR rotv"
  Demux1/31 -> BusCreator2/31  "PT IF WRL Trq_B2W"
  Demux1/32 -> BusCreator2/32  "PT IF WRL Trq_Drive"
  Demux1/36 -> BusCreator2/36  "PT IF WRR rot"
  Zero3/1 -> Bus Creator1/26, Bus Creator1/27
  Demux/4 -> Memory4/1, Discrete-Time Integrator7/1, Bus Creator1/37  "rotv RR"
  Zero2/1 -> Bus Creator1/19, Bus Creator1/20
  Zero1/1 -> Bus Creator1/5, Bus Creator1/4, Bus Creator1/12, Bus Creator1/14, Bus Creator1/13, Bus Creator1/11, Bus Creator1/10, Bus Creator1/9, Bus Creator1/8
  Demux1/20 -> BusCreator2/20  "PT IF WFL Trq_BrakeReg"
  Product2/1 -> Gain7/1
  Discrete-Time Integrator4/1 -> Bus Creator1/15  "PT WFL rot"
  Demux/2 -> Memory1/1, Discrete-Time Integrator5/1, Bus Creator1/23  "rotv FR"
  Discrete-Time Integrator7/1 -> Bus Creator1/36  "PtT WRR rot"
  Zero5/1 -> Bus Creator1/40, Bus Creator1/41, Bus Creator1/42
  Demux1/6 -> BusCreator2/6  "PT IF Trq_Supp2Bdy1 x"
  Demux1/41 -> BusCreator2/41  "PT IF WRR Trq_BrakeReg"
  BrakingTorques/1 -> Bus Selector2/1
  Operation Error/1 -> Bus Creator1/3
  Demux/3 -> Memory2/1, Discrete-Time Integrator6/1, Bus Creator1/30  "rotv RL"
  Memory1/1 -> Saturation1/1
  Ground4/1 -> Bus Creator1/6
  Bus Selector2/1 -> Product3/1  "<Brake IF Trq_WB FL>"
  Gain6/1 -> Bus Creator1/24
  Ignition/1 -> Bus Creator1/1  "PT Ignition"
  Memory2/1 -> Saturation2/1
  Saturation1/1 -> Product1/2
  Bus Selector2/3 -> Product2/1  "<Brake IF Trq_WB RL>"
  Gain7/1 -> Bus Creator1/31
  Demux/1 -> Memory3/1, Discrete-Time Integrator4/1, Bus Creator1/16  "rotv FL"
  Product4/1 -> Gain8/1
  Bus Creator1/1 -> Demux1/1
  Saturation2/1 -> Product2/2
  Product1/1 -> Gain6/1
  Bus Selector2/4 -> Product4/1  "<Brake IF Trq_WB RR>"
  Saturation3/1 -> Product3/2
  RotoWheelSpd/1 -> Demux/1
  AxlTrq/1 -> Demux2/1
  Demux2/1 -> Bus Creator1/18  "TrqDrv FL"
  Demux2/2 -> Bus Creator1/25  "TrqDrv FR"
  Demux2/3 -> Bus Creator1/32  "TrqDrv RL"
  Demux2/4 -> Bus Creator1/39  "TrqDrv RR"

== system CM13_2024a_MachE_for_UA_HIL/CarMaker_new/IPG Vehicle/Rototest and ORNL Interface/From Rototest ==
  Input : Inport
  Bus Creator : BusCreator  Inputs=30
  Bus Selector1 : BusSelector  OutputSignals=ActSpLF_rpm,ActSpRF_rpm,ActSpLR_rpm,ActSpRR_rpm
  Mux1 : Mux
  RotoTestEthRX : Subsystem  AncestorBlock=VSIGenLib/RotoTestEthRX
      mask Display:
      | color('white')
      | disp('RotTestEthTx')
      | port_label('output', 1, 'ID')
      | port_label('output', 2, 'ProtocolVer')
      | port_label('output', 3, 'ActTqLF (Nm)')
      | port_label('output', 4, 'RefRR_NmORrpm')
      | port_label('output', 5, 'ActTempLF (C)')
      | port_label('output', 6, 'ActTqRF (Nm)')
      | port_label('output', 7, 'ActSpRF (rpm)')
      | port_label('output', 8, 'ActTempRF (C)')
      | port_label('output', 9, 'ActTqLR (Nm)')
      | port_label('output', 10, 'ActSpLR (rpm)')
      | port_label('output', 11, 'ActTempLR (C)')
      | port_label('output', 12, 'ActTqRR (Nm)')
      | port_label('output', 13, 'ActSpRR (rpm)')
      | port_label('output', 14, 'ActTempRR (Nm)')
      | port_label('output', 15, 'RefLF (Nm)')
      | port_label('output', 16, 'RefRF (rpm)')
      | port_label('output', 17, 'RefLR (Nm)')
      | port_label('output', 18, 'RefRR (Nm)')
      | port_label('output', 19, 'UnitsStatusLF (enum)')
      | port_label('output', 20, 'UnitsStatusRF (enum)')
      | port_label('output', 21, 'UnitsStatusLR (enum)')
      | port_label('output', 22, 'UnitsStatusRR (enum)')
      | port_label('output', 23, 'WatchdogCnt (int)')
      | port_label('output', 24, 'FaultActive (enum)')
      | port_label('output', 25, 'WarningsActive (enum)')
      | port_label('output', 26, 'SpTqRR (enum)')
      | port_label('output', 27, 'SpTqLR (enum)')
      | port_label('output', 28, 'SpTqRF (enum)')
      | port_label('output', 29, 'SpTqLF (enum)')
      | port_label('output', 30, 'SystemActive (bool)')
  SpdAct : Outport
  AxlTrq : Outport  Port=2
  wires:
  RotoTestEthRX/8(ActTempRF_C) -> Bus Creator/8
  RotoTestEthRX/23(WatchdogCnt) -> Bus Creator/23
  RotoTestEthRX/18(RefRR_Nm) -> Bus Creator/18
  Mux1/1 -> SpdAct/1
  RotoTestEthRX/19(UnitsStatusLF) -> Bus Creator/19
  RotoTestEthRX/4(ActSpLF_rpm) -> Bus Creator/4
  Bus Creator/1 -> AxlTrq/1, Bus Selector1/1
  Bus Selector1/4 -> Mux1/4  "<ActSpRR_rpm>"
  RotoTestEthRX/24(FaultActive) -> Bus Creator/24
  RotoTestEthRX/22(UnitsStatusRR) -> Bus Creator/22
  Bus Selector1/3 -> Mux1/3  "<ActSpLR_rpm>"
  RotoTestEthRX/25(WarningsActive) -> Bus Creator/25
  Bus Selector1/1 -> Mux1/1  "<ActSpLF_rpm>"
  Bus Selector1/2 -> Mux1/2  "<ActSpRF_rpm>"
  RotoTestEthRX/5(ActTempLF_C) -> Bus Creator/5
  RotoTestEthRX/30(SystemActive) -> Bus Creator/30
  RotoTestEthRX/20(UnitsStatusRF) -> Bus Creator/20
  RotoTestEthRX/15(RefLF_Nm) -> Bus Creator/15
  RotoTestEthRX/16(RefRF_rpm) -> Bus Creator/16
  RotoTestEthRX/17(RefLR_Nm) -> Bus Creator/17
  RotoTestEthRX/2(ProtocolVer) -> Bus Creator/2
  RotoTestEthRX/7(ActSpRF_rpm) -> Bus Creator/7
  RotoTestEthRX/21(UnitsStatusLR) -> Bus Creator/21
  RotoTestEthRX/11(ActTempLR_C) -> Bus Creator/11
  RotoTestEthRX/1(ID) -> Bus Creator/1
  RotoTestEthRX/28(SpTqRF) -> Bus Creator/28
  RotoTestEthRX/29(SpTqLF) -> Bus Creator/29
  RotoTestEthRX/27(SpTqLR) -> Bus Creator/27
  RotoTestEthRX/26(SpTqRR) -> Bus Creator/26
  RotoTestEthRX/14(ActTempRR_Nm) -> Bus Creator/14
  RotoTestEthRX/3(ActTqLF_Nm) -> Bus Creator/3
  RotoTestEthRX/6(ActTqRF_Nm_) -> Bus Creator/6
  RotoTestEthRX/9(ActTqLR_Nm) -> Bus Creator/9
  RotoTestEthRX/13(ActSpRR_rpm) -> Bus Creator/13
  RotoTestEthRX/10(ActSpLR_rpm) -> Bus Creator/10
  RotoTestEthRX/12(ActTqRR_Nm) -> Bus Creator/12
  Input/1 -> RotoTestEthRX/1(Input)

== system CM13_2024a_MachE_for_UA_HIL/CarMaker_new/IPG Vehicle/Rototest and ORNL Interface/Get Wheel Spd Cmd Based on Wheel Dynamics ==
  BrakingTorques : Inport
  Trq_T2W : Inport  Port=2
  AxlTrq : Inport  Port=3
  MaxRegen : Inport  Port=4
  Saturation : Saturate  UpperLimit=100  LowerLimit=-100
  Saturation1 : Saturate  UpperLimit=300  LowerLimit=-300
  WheelSpdCmd : Subsystem
  Whl Dynamics & Format CM Powertrain Signal : Subsystem
  WhlSpdCmd : Outport
  wires:
  Whl Dynamics & Format CM Powertrain Signal/1(PowerTrainOutIdeal) -> WheelSpdCmd/1(In1)
  BrakingTorques/1 -> Whl Dynamics & Format CM Powertrain Signal/1(BrakingTorques)
  Trq_T2W/1 -> Whl Dynamics & Format CM Powertrain Signal/2(Trq_T2W)
  MaxRegen/1 -> Whl Dynamics & Format CM Powertrain Signal/4(MaxRegen)
  [SimOmega] -> Saturation/1
  Saturation/1 -> WhlSpdCmd/1
  AxlTrq/1 -> Whl Dynamics & Format CM Powertrain Signal/3(AxlTrq)

== system CM13_2024a_MachE_for_UA_HIL/CarMaker_new/IPG Vehicle/Rototest and ORNL Interface/RotoTrqPreprocess ==
  AxleTrqRaw : Inport
  Bus Selector1 : BusSelector  OutputSignals=ActTqLF_Nm_,ActTqRF_Nm_,ActTqLR_Nm_,ActTqRR_Nm
  Compare To Constant : simulink/Logic and Bit Operations/Compare To Constant  relop=>=  const=-15  OutDataTypeStr=boolean
  Compare To Constant1 : simulink/Logic and Bit Operations/Compare To Constant  relop=<=  const=0  OutDataTypeStr=boolean
  Data Type Conversion{1..4} (4 alike) : DataTypeConversion  OutDataTypeStr=double  SaturateOnIntegerOverflow=off  RndMeth=Floor
  FirstOrderFilterTau{,1..3} (4 alike) : VSIGenLib/FirstOrderFilterTau  SystemSampleTime=-1  VariantActivationTime=update diagram  AllowFlexibleInterface=on  Latency=0  AutoFrameSizeCalculation=off
  Ground : Ground
  Logical Operator : Logic  AllPortsSameDT=off  OutDataTypeStr=boolean
  ManualTrq_Nm : Constant  Value=0
  Mux : Mux
  Mux1 : Mux
  SatTrq : Saturate  UpperLimit=2800  LowerLimit=-2800
  Tau : Constant  Value=0.01
  TorqueIn : Switch  Criteria=u2 > Threshold  SaturateOnIntegerOverflow=off  InputSameDT=off
  "TorqueIn " : Switch  Criteria=u2 > Threshold  SaturateOnIntegerOverflow=off  InputSameDT=off
  AxleTrqRoto : Outport
  AxleTrqVeh : Outport  Port=2
  wires:
  Mux/1 -> AxleTrqRoto/1, TorqueIn/1
  ManualTrq_Nm/1 -> Mux1/4, Mux1/3, Mux1/2, Mux1/1
  Tau/1 -> FirstOrderFilterTau/2, FirstOrderFilterTau1/2, FirstOrderFilterTau2/2, FirstOrderFilterTau3/2
  Ground/1 -> "TorqueIn "/1
  Logical Operator/1 -> "TorqueIn "/2
  Data Type Conversion4/1 -> Mux/4  "RR"
  Data Type Conversion3/1 -> Mux/3  "LR"
  Mux1/1 -> TorqueIn/3
  [Switch] -> TorqueIn/2
  Bus Selector1/4 -> FirstOrderFilterTau3/1  "<ActTqRR_Nm>"
  Compare To Constant/1 -> Logical Operator/1
  Bus Selector1/3 -> FirstOrderFilterTau2/1  "<ActTqLR_Nm_>"
  Bus Selector1/2 -> FirstOrderFilterTau1/1  "<ActTqRF_Nm_>"
  TorqueIn/1 -> SatTrq/1
  "TorqueIn "/1 -> AxleTrqVeh/1  "Trq"
  FirstOrderFilterTau1/1 -> Data Type Conversion2/1
  Data Type Conversion2/1 -> Mux/2  "RF"
  AxleTrqRaw/1 -> Bus Selector1/1
  FirstOrderFilterTau/1 -> Data Type Conversion1/1
  FirstOrderFilterTau3/1 -> Data Type Conversion4/1
  Bus Selector1/1 -> FirstOrderFilterTau/1  "<ActTqLF_Nm_>"
  Compare To Constant1/1 -> Logical Operator/2
  SatTrq/1 -> "TorqueIn "/3, Compare To Constant1/1, Compare To Constant/1
  FirstOrderFilterTau2/1 -> Data Type Conversion3/1
  Data Type Conversion1/1 -> Mux/1  "LF"

== system CM13_2024a_MachE_for_UA_HIL/CarMaker_new/IPG Vehicle/Rototest and ORNL Interface/Subsystem2 ==
  AxlTorq : Inport
  BusCreator1 : BusCreator  Inputs=16
  BusCreator2 : BusCreator  Inputs=16
  Constant : Constant  Value=0
  Constant1 : Constant  Value=0
  Demux : Demux  Outputs=16
      settings: DisplayOption=none
  Terminator : Terminator
  Zero1 : Constant  Value=0
  Zero2 : Constant  Value=0
  Zero5 : Constant  Value=0
  BrakeUpd : Outport
  wires:
  Demux/9 -> BusCreator1/9  "Brake IF Trq_Reg_trg FL"
  Demux/6 -> BusCreator1/6  "Brake IF Trq_PB FR"
  Constant1/1 -> BusCreator2/1, BusCreator2/2  "Brake IF Trq_WB FL"
  Demux/14 -> BusCreator1/14  "Brake IF Trq_DriveSrc_trg d1"
  Zero2/1 -> BusCreator2/16, BusCreator2/15, BusCreator2/14, BusCreator2/13  "Brake IF Trq_DriveSrc_trg d3"
  Demux/11 -> BusCreator1/11  "Brake IF Trq_Reg_trg RL"
  Demux/15 -> BusCreator1/15  "Brake IF Trq_DriveSrc_trg d2"
  Demux/2 -> BusCreator1/2  "Brake IF Trq_WB FR"
  Demux/16 -> BusCreator1/16  "Brake IF Trq_DriveSrc_trg d3"
  Zero1/1 -> BusCreator2/12, BusCreator2/11, BusCreator2/10, BusCreator2/9  "Brake IF Trq_Reg_trg RR"
  Demux/4 -> BusCreator1/4  "Brake IF Trq_WB RR"
  Demux/3 -> BusCreator1/3  "Brake IF Trq_WB RL"
  Constant/1 -> BusCreator2/4, BusCreator2/3  "Brake IF Trq_WB RL"
  BusCreator1/1 -> BrakeUpd/1
  Demux/1 -> BusCreator1/1  "Brake IF Trq_WB FL"
  Demux/8 -> BusCreator1/8  "Brake IF Trq_PB RR"
  Demux/10 -> BusCreator1/10  "Brake IF Trq_Reg_trg FR"
  BusCreator2/1 -> Demux/1
  Demux/13 -> BusCreator1/13  "Brake IF Trq_DriveSrc_trg d0"
  Demux/5 -> BusCreator1/5  "Brake IF Trq_PB FL"
  Demux/7 -> BusCreator1/7  "Brake IF Trq_PB RL"
  Zero5/1 -> BusCreator2/8, BusCreator2/7, BusCreator2/6, BusCreator2/5  "Brake IF Trq_PB RR"
  Demux/12 -> BusCreator1/12  "Brake IF Trq_Reg_trg RR"
  AxlTorq/1 -> Terminator/1

== system CM13_2024a_MachE_for_UA_HIL/CarMaker_new/IPG Vehicle/Rototest and ORNL Interface/To Rototest with Band-Aid ==
  note: Torque Model: Low speed
      | Speed Model: Normal speed
  note: OutMode = 0 is Torque
      | OutMode = 1 is Speed
  note: Switch = 0 Overides
      | Switch = 1 Model
      | With Auto_MasterSW, User need to TurnOn_SW first
  SpeedCmd_rps : Inport
  AxleTrq_roto_Nm : Inport  Port=2
  BRAKE_PRESSED : Inport  Port=3
  Vehicle_Speed_kph : Inport  Port=4
  SpdAct : Inport  Port=5
  AND : Logic  Commented=on  IconShape=distinctive  AllPortsSameDT=off  OutDataTypeStr=boolean
  Auto_MasterSW : Subsystem  Commented=on
  Band-Aid : Subsystem
  Demux : Demux
  Demux1 : Demux
  Demux2 : Demux
  Logging : Subsystem  Commented=on
  MasterSw : Constant  Value=0
  Mode Override : Subsystem
  ModeOut : Switch  Criteria=u2 > Threshold  SaturateOnIntegerOverflow=off  InputSameDT=off
  ModeSwitch : MultiPortSwitch  DataPortOrder=Zero-based contiguous  Inputs=2  zeroidx=on  SaturateOnIntegerOverflow=off  InputSameDT=off
  Mux2 : Mux
  Mux4 : Mux
  Mux5 : Mux
  RateLimSpd : RateLimiter  RisingSlewLimit=500  FallingSlewLimit=-500  SampleTimeMode=inherited
  RotoTestEthTx : Subsystem  AncestorBlock=VSIGenLib/RotoTestEthTx
      mask Display:
      | color('white')
      | disp('RotTestEthTx')
      | port_label('input', 1, 'RefLF_NmORrpm')
      | port_label('input', 2, 'RefRF_NmORrpm')
      | port_label('input', 3, 'RefLR_NmORrpm')
      | port_label('input', 4, 'RefRR_NmORrpm')
      | port_label('input', 5, 'SqTrRR')
      | port_label('input', 6, 'SqTrLR')
      | port_label('input', 7, 'SqTrRF')
      | port_label('input', 8, 'SqTrLF')
      | port_label('input', 9, 'SystemActive')
      | port_label('output', 1, 'Status (bool)')
      | port_label('output', 2, 'Sent Bytes (int)')
  SatSpd : Saturate  UpperLimit=2000  LowerLimit=0
  SpeedOut : Switch  Criteria=u2 > Threshold  SaturateOnIntegerOverflow=off  InputSameDT=off
  SteeringSystem : Subsystem
  SystemActive : Constant  Value=0  OutDataTypeStr=uint8
  Terminator : Terminator  Commented=on
  Terminator1 : Terminator  Commented=on
  TrqSpd Override : Subsystem
  ZeroTorque : Constant  Value=0  OutDataTypeStr=uint8
  rads2rpm : Gain  Gain=9.5492965964254
  Out1 : Outport
  AutoMasterSW_Signal : Outport  Port=2
  tag scope: Switch=global
  wires:
  Mux4/1 -> ModeSwitch/2
  Demux/3 -> Mux2/3  "LRIn"
  Demux1/4 -> RotoTestEthTx/4(RefRR_NmORrpm)
  Demux/2 -> Mux2/2  "RFIn"
  MasterSw/1 -> AutoMasterSW_Signal/1, [Switch]
  TrqSpd Override/1(Ovr) -> SpeedOut/3
  ZeroTorque/1 -> Mux4/2, Mux4/3, Mux4/4, Mux4/1
  Demux/1 -> Mux2/1  "LFIn"
  SpeedOut/1 -> RateLimSpd/1
  RateLimSpd/1 -> SatSpd/1
  rads2rpm/1 -> Demux/1
  ModeSwitch/1 -> Demux1/1
  Demux/4 -> Mux2/4  "RRIn"
  Band-Aid/1(OutMode) -> Mux5/4, Mux5/3, Mux5/2, Mux5/1, ModeSwitch/1
  ModeOut/1 -> Demux2/1
  [Switch] -> SpeedOut/2
  SatSpd/1 -> ModeSwitch/3  "Spd"
  [Switch] -> ModeOut/2
  Mux5/1 -> ModeOut/1
  Demux2/1 -> RotoTestEthTx/5(SpTqRR)
  Demux1/3 -> RotoTestEthTx/3(RefLR_NmORrpm)
  Demux2/3 -> RotoTestEthTx/7(SpTqRF)
  Demux2/2 -> RotoTestEthTx/6(SpTqLR)
  SystemActive/1 -> RotoTestEthTx/9(SystemActive)
  RotoTestEthTx/1(Output) -> Out1/1  "ByteSend"
  Demux1/1 -> RotoTestEthTx/1(RefLF_NmORrpm)
  Demux1/2 -> RotoTestEthTx/2(RefRF_NmORrpm)
  Demux2/4 -> RotoTestEthTx/8(SpTqLF)
  SpeedCmd_rps/1 -> rads2rpm/1
  Mode Override/1(Ovr) -> ModeOut/3
  AxleTrq_roto_Nm/1 -> Band-Aid/2(InTrq_Nm)
  Mux2/1 -> Band-Aid/1(InSpd_rpm)
  Band-Aid/2(OutSpd_rpm) -> SpeedOut/1
  BRAKE_PRESSED/1 -> Band-Aid/3(BRAKE_PRESSED)
  Vehicle_Speed_kph/1 -> Band-Aid/4(VehSpd_kph)
  Auto_MasterSW/1(Auto_MasterSW) -> Terminator/1, AND/1  "AutoMasterSW_sig"
  AND/1 -> Terminator1/1  "MSW_sig"
  SpdAct/1 -> Auto_MasterSW/1(SpdAct)

== system CM13_2024a_MachE_for_UA_HIL/CarMaker_new/IPG Vehicle/SUMO Spd/dSPACE TCP Out ==
  ByteSend : Inport
  nMsgSend : Inport  Port=2
  sendTrigger : Inport  Port=3
  Constant1 : Constant  Value=0
  Data Type Conversion4 : DataTypeConversion  SaturateOnIntegerOverflow=off  RndMeth=Floor
  Display7 : Display
  Transmit_Out [TCP Ref Speed]1 : dsmpblib/Data Outport  Priority=-10000
      settings: SourceProductName=dSPACE Model Interface Package for Simulink (MIPS)
  switch for 0.1 send out : Switch  Criteria=u2 > Threshold  SaturateOnIntegerOverflow=off  InputSameDT=off
  wires:
  Constant1/1 -> switch for 0.1 send out/3
  nMsgSend/1 -> Data Type Conversion4/1
  Data Type Conversion4/1 -> switch for 0.1 send out/1, Display7/1
  switch for 0.1 send out/1 -> Transmit_Out [TCP Ref Speed]1/2  "sendByteSize_RealSimPack"
  ByteSend/1 -> Transmit_Out [TCP Ref Speed]1/1
  sendTrigger/1 -> switch for 0.1 send out/2

== system CM13_2024a_MachE_for_UA_HIL/CarMaker_new/IPG Vehicle/Steering Angle HIL/Steering Override ==
  note: IPG
      | 	positive left turn, negative right turn
  note: SteerOverrideSwitch
      | 0: use IPG steer
      | 1: use CAN steer
      | 2: use manual input
  SteerAngCAN_in : Inport
  <VhclCtrl Steering Ang> : Inport  Port=2
  Gain : Gain
  Gain1 : Gain  Gain=pi/180
  Multiport Switch : MultiPortSwitch  DataPortOrder=Zero-based contiguous  zeroidx=on  SaturateOnIntegerOverflow=off  InputSameDT=off
  SteerManual : Constant  Value=0
  SteerOverrideSwitch : Constant  Value=0
  VhclCtrl Steering Ang : Outport
  wires:
  SteerManual/1 -> Gain/1
  Gain1/1 -> Multiport Switch/3  "SteerAngCAN_rad"
  Gain/1 -> Multiport Switch/4
  SteerOverrideSwitch/1 -> Multiport Switch/1
  Multiport Switch/1 -> VhclCtrl Steering Ang/1  "VhclCtrl Steering Ang"
  <VhclCtrl Steering Ang>/1 -> Multiport Switch/2
  SteerAngCAN_in/1 -> Gain1/1

== system CM13_2024a_MachE_for_UA_HIL/FIXS/RealSim Core/RealSim CreatBus/rgba2uint ==
  In1 : Inport
  Divide : Product  Inputs=**
  Sum of Elements : Sum  Inputs=+
  rgba bit operation : Constant  Value=[2^24,2^16,2^8,2^0]
  Out1 : Outport
  wires:
  Sum of Elements/1 -> Out1/1
  rgba bit operation/1 -> Divide/2
  In1/1 -> Divide/1
  Divide/1 -> Sum of Elements/1

== system CM13_2024a_MachE_for_UA_HIL/FIXS1/RealSim Translate CM Signal to Bus as Feedback to SUMO//VISSIM/RealSim CreatBus/rgba2uint ==
  In1 : Inport
  Divide : Product  Inputs=**
  Sum of Elements : Sum  Inputs=+
  rgba bit operation : Constant  Value=[2^24,2^16,2^8,2^0]
  Out1 : Outport
  wires:
  Divide/1 -> Sum of Elements/1
  In1/1 -> Divide/1
  rgba bit operation/1 -> Divide/2
  Sum of Elements/1 -> Out1/1

== system CM13_2024a_MachE_for_UA_HIL/RealSim1/ToRealSim/RealSim CreatBus/rgba2uint ==
  In1 : Inport
  Divide : Product  Inputs=**
  Sum of Elements : Sum  Inputs=+
  rgba bit operation : Constant  Value=[2^24,2^16,2^8,2^0]
  Out1 : Outport
  wires:
  Sum of Elements/1 -> Out1/1
  rgba bit operation/1 -> Divide/2
  In1/1 -> Divide/1
  Divide/1 -> Sum of Elements/1

== system CM13_2024a_MachE_for_UA_HIL/RealSim2/ToRealSim/RealSim CreatBus/rgba2uint ==
  In1 : Inport
  Divide : Product  Inputs=**
  Sum of Elements : Sum  Inputs=+
  rgba bit operation : Constant  Value=[2^24,2^16,2^8,2^0]
  Out1 : Outport
  wires:
  Divide/1 -> Sum of Elements/1
  In1/1 -> Divide/1
  rgba bit operation/1 -> Divide/2
  Sum of Elements/1 -> Out1/1

== system CM13_2024a_MachE_for_UA_HIL/Vehicle Under Test2/Environment/Ground Feedback/3D Engine ==
  Friction : Inport
  Ground Z Level : Inport  Port=2
  Bus Creator : BusCreator  Inputs=4
  Bus Creator2 : BusCreator  Inputs=4
  Bus Creator3 : BusCreator  Inputs=2
  Bus Selector : BusSelector  OutputSignals=HitLoc
  Data Type Conversion : DataTypeConversion  SaturateOnIntegerOverflow=off  RndMeth=Floor
  Demux : Demux
  Demux1 : Demux
  Passenger Vehicle Ray Trace Set : sim3dlib/Vehicle Terrain Sensor  Priority=1  ActorTag=SimulinkVehicle1  VehExtEn=Constant  TireRadiiExt=Constant  VehCntrLngthVal=0  TireRadiiVal=0  VehRayLngth=10  LfRayLngth=20  RfRayLngth=20  LrRayLngth=20  RrRayLngth=20  VehRayOffset=0  LfRayOffset=-1  RfRayOffset=-1  LrRayOffset=-1  RrRayOffset=-1  VehEn=on  LfEn=on  RfEn=on  LrEn=on  RrEn=on  DbgEn=off  Ts=.03  aMode=aMode
  Rate Transition : RateTransition
  Reshape10 : Reshape  OutputDimensionality=Row vector (2-D)
  Selector1 : Selector  InputPortWidth=5  IndexOptions=Index vector (dialog)  Indices=[2:5]  OutputSizes=1
  Signal Specification : SignalSpecification  Unit=m
  Signal Specification1 : SignalSpecification  Unit=1
  Terminator : Terminator
  Terminator1 : Terminator
  Terminator2 : Terminator
  Zend Select : Selector  NumberOfDimensions=2  InputPortWidth=3  IndexOptions=Select all,Index vector (dialog)  Indices=[1 3],3  OutputSizes=1,1
  Ground : Outport  VectorParamsAs1DForOutWhenUnconnected=off
  wires:
  Selector1/1 -> Rate Transition/1
  Zend Select/1 -> Reshape10/1
  Bus Selector/1 -> Zend Select/1  "<HitLoc>"
  Passenger Vehicle Ray Trace Set/2 -> Terminator1/1
  Passenger Vehicle Ray Trace Set/3 -> Terminator2/1
  Reshape10/1 -> Selector1/1
  Passenger Vehicle Ray Trace Set/1 -> Bus Selector/1
  Rate Transition/1 -> Data Type Conversion/1
  Demux/2 -> Bus Creator/2  "G_FR_z"
  Demux/1 -> Bus Creator/1  "G_FL_z"
  Demux/4 -> Bus Creator/4  "G_RR_z"
  Demux/3 -> Bus Creator/3  "G_RL_z"
  Signal Specification/1 -> Demux/1
  Signal Specification1/1 -> Demux1/1
  Demux1/1 -> Bus Creator2/1  "mu_FL"
  Bus Creator/1 -> Bus Creator3/1  "z"
  Demux1/3 -> Bus Creator2/3  "mu_RL"
  Demux1/4 -> Bus Creator2/4  "mu_RR"
  Demux1/2 -> Bus Creator2/2  "mu_FR"
  Bus Creator2/1 -> Bus Creator3/2  "mu"
  Bus Creator3/1 -> Ground/1
  Friction/1 -> Signal Specification1/1
  Data Type Conversion/1 -> Signal Specification/1
  Ground Z Level/1 -> Terminator/1

== system CM13_2024a_MachE_for_UA_HIL/Vehicle Under Test2/Environment/Ground Feedback/Constant ==
  Friction : Inport
  Ground Z Level : Inport  Port=2
  Bus Creator : BusCreator  Inputs=4
  Bus Creator2 : BusCreator  Inputs=4
  Bus Creator3 : BusCreator  Inputs=2
  Demux : Demux
  Demux1 : Demux
  Signal Specification : SignalSpecification  Unit=m
  Signal Specification1 : SignalSpecification  Unit=1
  Ground : Outport  VectorParamsAs1DForOutWhenUnconnected=off
  wires:
  Ground Z Level/1 -> Signal Specification/1
  Signal Specification/1 -> Demux/1
  Demux/4 -> Bus Creator/4  "G_RR_z"
  Demux/1 -> Bus Creator/1  "G_FL_z"
  Demux/3 -> Bus Creator/3  "G_RL_z"
  Demux/2 -> Bus Creator/2  "G_FR_z"
  Bus Creator/1 -> Bus Creator3/1  "z"
  Demux1/3 -> Bus Creator2/3  "mu_RL"
  Demux1/4 -> Bus Creator2/4  "mu_RR"
  Demux1/1 -> Bus Creator2/1  "mu_FL"
  Demux1/2 -> Bus Creator2/2  "mu_FR"
  Bus Creator2/1 -> Bus Creator3/2  "mu"
  Friction/1 -> Signal Specification1/1
  Signal Specification1/1 -> Demux1/1
  Bus Creator3/1 -> Ground/1
